simulink model "MinSeg_Lab2_Gyroscope3"  (R2014b)
settings: Solver=FixedStepDiscrete  StartTime=0.0  StopTime=inf  FixedStep=0.03  RelTol=1e-3
settings Model: SimulationMode=external  ExtModeTrigDuration=2  Creator=hrlin  LastModifiedBy=lq561d
settings OptimizationCC: OptimizeModelRefInitCode=on  LifeSpan=1
settings DebuggingCC: SolverPrmCheckMsg=none
settings HardwareCC: ProdBitPerInt=16  ProdBitPerPointer=8  ProdIntDivRoundTo=Zero  ProdEndianess=LittleEndian  ProdWordSize=8  ProdHWDeviceType=Atmel->AVR
settings RTWCC: SystemTargetFile=realtime.tlc  GenerateMakefile=off  TemplateMakefile=realtime.tmf  Description=Run on Target Hardware  RTWVerbose=off  ProcessScript=realtime_make_rtw_hook
settings STFCustomTargetCC: TargetLibSuffix=.a  GenerateSampleERTMain=on  ERTCustomFileBanners=on  SupportNonInlinedSFcns=off  SupportVariableSizeSignals=on  MATLABClassNameForMDSCustomization=Simulink.SoftwareTarget.ERTCustomization  GRTInterface=off  SystemTargetFile=realtime.tlc
settings ERTTargetCC: GenerateSampleERTMain=on  ParMdlRefBuildCompliant=off  CompOptLevelCompliant=off  ConcurrentExecutionCompliant=off  CombineOutputUpdateFcns=off  ERTFirstTimeCompliant=off  SupportContinuousTime=on  SupportVariableSizeSignals=on  ModelStepFunctionPrototypeControlCompliant=off  CPPClassGenCompliant=off  ExtModeTransport=3  ExtModeMexFile=ext_serial_win32_comm  ExtModeMexArgs=0 1 9600  InlinedParameterPlacement=NonHierarchical  ERTSrcFileBannerTemplate=realtime_code_template.cgt  ERTHdrFileBannerTemplate=realtime_code_template.cgt  ERTDataSrcFileTemplate=realtime_code_template.cgt  ERTDataHdrFileTemplate=realtime_code_template.cgt  ERTCustomFileTemplate=realtime_file_process.tlc

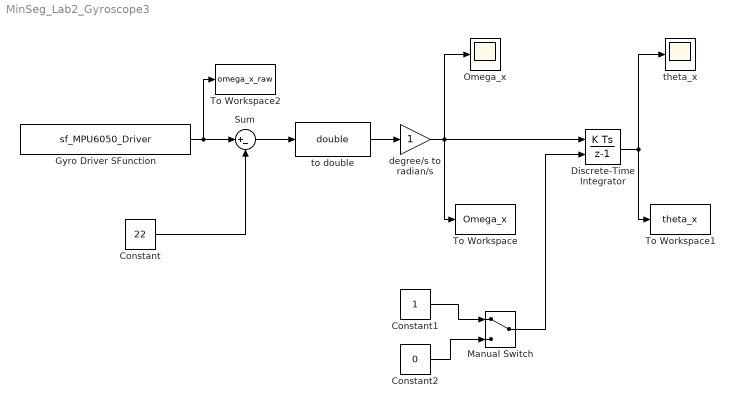
== system MinSeg_Lab2_Gyroscope3 ==
  Constant : Constant  Value=22
  Constant1 : Constant
  Constant2 : Constant  Value=0
  Discrete-Time Integrator : DiscreteIntegrator  ExternalReset=either  InitialConditionSetting=State (most efficient)  SampleTime=-1
  Gyro Driver SFunction : S-Function  InitFcn=try, set_param(gcb,'FunctionName','sf_MPU6050_Driver'), end  FunctionName=sf_MPU6050_Driver  SFunctionModules=sf_MPU6050_Driver_wrapper  EnableBusSupport=off  mask(S-Function Builder){}
      mask help: Simulink:masks:SFunctionBuilder_MD
      mask init:
      | val = [[.9  0.75 0.75 1 1 .9 .9 1]',[1 1 0.75 0.75 .9 .9 1 .9]'];try , sys = get_param(gcb,'SfunBuilderFcnName');if isempty(sys), sys = get_param(gcb,'FunctionName'); end,catch, sys = get_param(gcb,'FunctionName'); end
      settings: CopyFcn=set_param(gcbh,'LinkStatus','none')  PreSaveFcn=try, set_param(gcb,'FunctionName','sf_MPU6050_Driver'), end  OpenFcn=sfunctionwizard(gcbh)
      mask Display: plot(val(:,1),val(:,2)),disp(sys), port_label('output',1,'x_vel')
  Manual Switch : ManualSwitch
  Omega_x : Scope
      settings: YMin=-2  YMax=14
  Sum : Sum  Inputs=|+-
  To Workspace : ToWorkspace  VariableName=Omega_x  SampleTime=-1
  To Workspace1 : ToWorkspace  VariableName=theta_x  SampleTime=-1
  To Workspace2 : ToWorkspace  VariableName=omega_x_raw  SampleTime=-1
  "degree/s to radian/s " : Gain
  theta_x : Scope
      settings: YMin=69  YMax=72
  to double : DataTypeConversion  OutDataTypeStr=double
  wires:
  Discrete-Time Integrator/1 -> To Workspace1/1, theta_x/1
  Gyro Driver SFunction/1 -> To Workspace2/1, Sum/1
  Constant/1 -> Sum/2
  Constant1/1 -> Manual Switch/1
  Constant2/1 -> Manual Switch/2
  Manual Switch/1 -> Discrete-Time Integrator/2
  Sum/1 -> to double/1
  to double/1 -> "degree/s to radian/s "/1
  "degree/s to radian/s "/1 -> To Workspace/1, Omega_x/1, Discrete-Time Integrator/1
